simulink model "RM3"  (R2014b)
settings: Solver=ode4  StartTime=0  StopTime=200  FixedStep=0.001  RelTol=1e-3
values from neighbouring files (symbols this model uses):
  ptosim = ptoSimClass('Complex_Hydraulic')    [ptoSimInputFile.m]
undefined symbols (not defined in the file or in its folder): body, constraint, pto
libraries: PTOSim_Lib x6, WECSim_Lib x5
settings Model: Creator=mlawson  LastModifiedBy=rso
settings SolverCC: AlgebraicLoopSolver=LineSearch
settings DataIOCC: LimitDataPoints=off  SaveOutput=off  SaveTime=off
settings DebuggingCC: UnderspecifiedInitializationDetection=Classic  MergeDetectMultiDrivingBlocksExec=none  StateNameClashWarn=warning
settings ExplorerConfigSet: InternalSimMechanicsExplorerSettings="<ExplorerConfiguration><canonicalview>default</canonicalview><TilePanel><TileInfo><Tiles Columns=\"1\" Count=\"1\" Rows=\"1\"><Column Left=\"2\" Weight=\"1\"/><Column Left=\"1335\"/><Row Top=\"2\" Weight=\"1\"/><Row Top=\"911\"/><Tile Height=\"1\" Width=\"1\" X=\"0\" Y=\"0\"/></Tiles></TileInfo><SceneInfo><SceneViewer><BGColor><R>0.60000002384185791</R><G>0.60000002384185791</G><B>0.60000002384185791</B></BGColor><Camera><Position><X>365.37645888990272</X><Y>-369.82486814446582</Y><Z>359.64809521743916</Z></Position><Center><X>-6.7351450971904585</X><Y>2.2867358426280204</Y><Z>-12.463508769654169</Z></Center><Up><X>-0.40824829046386307</X><Y>0.40824829046386307</Y><Z>0.81649658092772615</Z></Up><Left>-57.820127362122818</Left><Right>57.820127362122818</Right><Bottom>-38.308817187253304</Bottom><Top>38.308817187253304</Top></Camera></SceneViewer></SceneInfo></TilePanel></ExplorerConfiguration>"

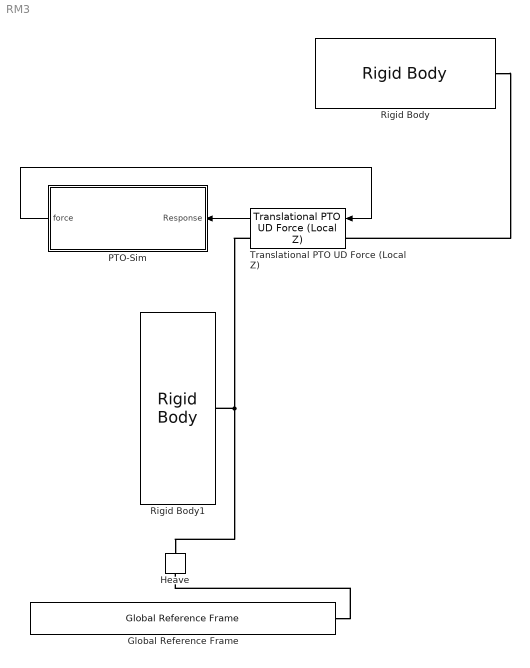
== system RM3 ==
  Global Reference Frame : WECSim_Lib/Frames/Global Reference Frame  waves=waves  simu=simu
  Heave : WECSim_Lib/Constraints/Heave  constraint=constraint(1)
      settings: AttributesFormatString=%<constraint>
  PTO-Sim : Subsystem  mask(PTO-Sim){ptoSim=0}
      mask prompts: ptoSim "PTO-Sim"
  Rigid Body : WECSim_Lib/Body Elements/Rigid Body  body=body(1)
      settings: AttributesFormatString=%<body>
  Rigid Body1 : WECSim_Lib/Body Elements/Rigid Body  body=body(2)
      settings: AttributesFormatString=%<body>
  Translational PTO UD Force (Local Z) : WECSim_Lib/PTOs/Translational PTO UD Force  (Local Z)  pto=pto(1)
      settings: AttributesFormatString=%<pto>
  wires:
  Translational PTO UD Force (Local Z)/1 -> PTO-Sim/1(Response)
  PTO-Sim/1(force) -> Translational PTO UD Force (Local Z)/1
  connections:
  Global Reference Frame/RConn1 -- Heave/LConn1
  Translational PTO UD Force (Local Z)/RConn1 -- Rigid Body1/RConn1 -- Heave/RConn1
  Rigid Body/RConn1 -- Translational PTO UD Force (Local Z)/LConn1

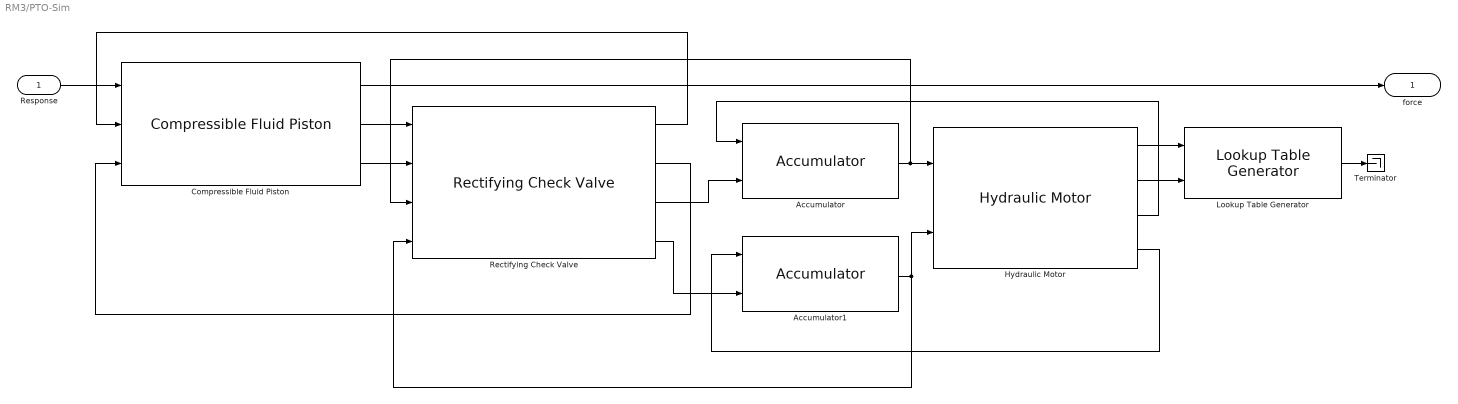
== system RM3/PTO-Sim ==
  Response : Inport
  Accumulator : PTOSim_Lib/Hydraulic/Accumulator  ptosim=ptosim.accum(1)
  Accumulator1 : PTOSim_Lib/Hydraulic/Accumulator  ptosim=ptosim.accum(2)
  Compressible Fluid Piston : PTOSim_Lib/Hydraulic/Compressible Fluid Piston  ptosim=ptosim.piston
  "Hydraulic Motor " : PTOSim_Lib/Hydraulic/Hydraulic Motor   ptosim=ptosim.motor
  Lookup Table Generator : PTOSim_Lib/Rotary Generator/Lookup Table  Generator  ptosim=ptosim.gen
  Rectifying Check Valve : PTOSim_Lib/Hydraulic/Rectifying Check Valve  ptosim=ptosim.valve
  Terminator : Terminator
  force : Outport
  wires:
  Response/1 -> Compressible Fluid Piston/1
  Compressible Fluid Piston/1 -> force/1
  "Hydraulic Motor "/1 -> Lookup Table Generator/1
  "Hydraulic Motor "/2 -> Lookup Table Generator/2
  "Hydraulic Motor "/3 -> Accumulator/1
  "Hydraulic Motor "/4 -> Accumulator1/1
  Lookup Table Generator/1 -> Terminator/1
  Accumulator/1 -> Rectifying Check Valve/3, "Hydraulic Motor "/1
  Accumulator1/1 -> "Hydraulic Motor "/2, Rectifying Check Valve/4
  Compressible Fluid Piston/2 -> Rectifying Check Valve/1
  Rectifying Check Valve/1 -> Compressible Fluid Piston/2
  Rectifying Check Valve/2 -> Compressible Fluid Piston/3
  Rectifying Check Valve/3 -> Accumulator/2
  Rectifying Check Valve/4 -> Accumulator1/2
  Compressible Fluid Piston/3 -> Rectifying Check Valve/2
